simulink model "wireless_signals_routing"  (R2021a)
settings: Solver=VariableStepAuto  StartTime=0.0  StopTime=10.0  RelTol=1e-3
libraries: simulink x1
settings Model: Creator=Acer  LastModifiedBy=Acer

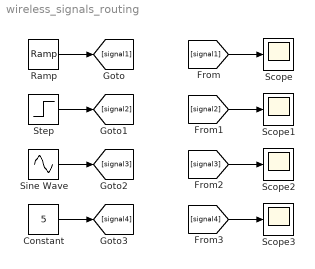
== system wireless_signals_routing ==
  Constant : Constant  Value=5
  Ramp : simulink/Sources/Ramp  slope=1  start=0  InitialOutput=0
  Scope{,1..3} (4 alike) : Scope
  Sine Wave : Sin  SampleTime=0
  Step : Step  SampleTime=0
  wires:
  Ramp/1 -> [signal1]
  [signal1] -> Scope/1
  Step/1 -> [signal2]
  [signal2] -> Scope1/1
  Sine Wave/1 -> [signal3]
  [signal3] -> Scope2/1
  Constant/1 -> [signal4]
  [signal4] -> Scope3/1
